simulink model "lab0_model_est"  (R2024b)
settings: Solver=ode45  StartTime=0.0  StopTime=sIn.t_sim  RelTol=1e-3
values from neighbouring files (symbols this model uses):
  PID = computePIDGains(8, 0.15, 0.1, plant.Ps, "PID")    [lab0_startup.m]
undefined symbols (not defined in the file or in its folder): degs2rpm, filt, gbox, rpm2degs, sens, sIn
libraries: simulink x2, simulink_extras x1
settings Model: Creator=pries  LastModifiedBy=pries
settings DataIOCC: ReturnWorkspaceOutputs=off

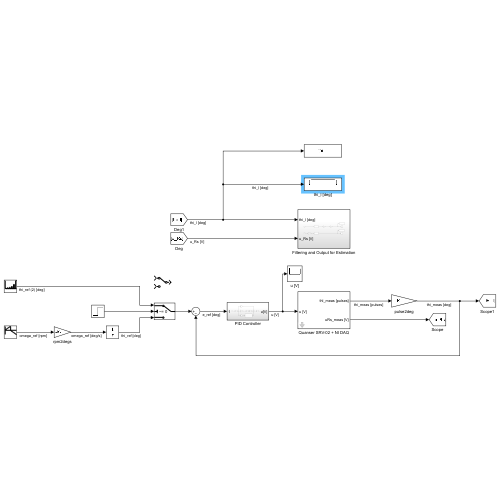
[thumbnail: Simulink's stored preview of the top-level diagram]
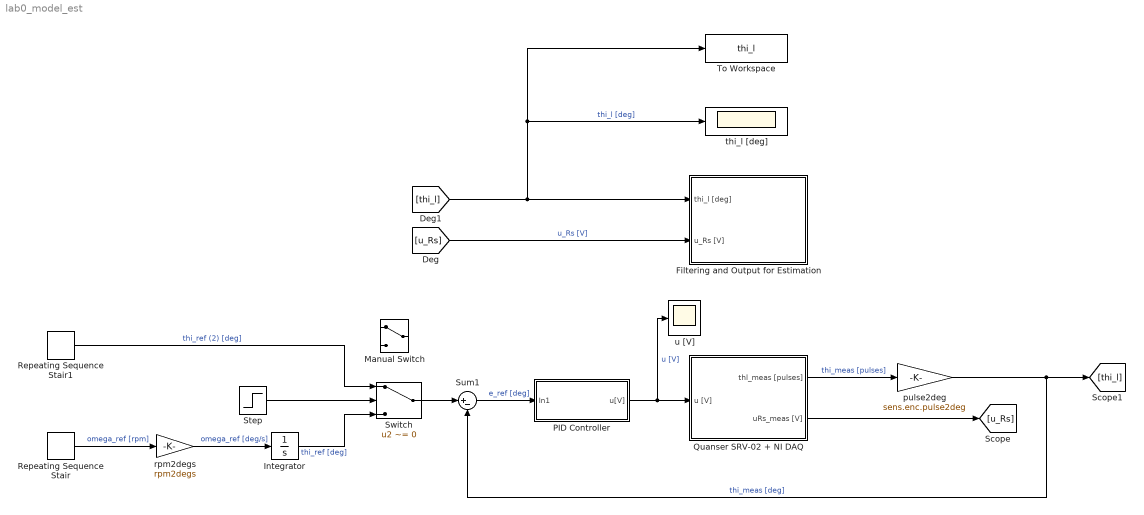
== system lab0_model_est ==
  Filtering and Output for Estimation : Subsystem
  Integrator : Integrator
  Manual Switch : ManualSwitch
  PID Controller : Subsystem
  Quanser SRV-02 + NI DAQ : Subsystem  mask(Quanser SRV-02 (with inertial load) + NI DAQ){Ts=0.001, fricType=Coulomb + viscous}
      mask prompts: Ts "NI DAQ Sample Time:"; fricType "Friction model"
      mask help: Quanser SRV-02 (with inertial load) + NI DAQ model.
      mask init:
      | %%  Sensors data
      | 
      | %   shunt resistor
      | sens.curr.Rs = 0.5;                         %   resistance [Ohm]   
      | sens.curr.uRs_std = 0.01;                   %   voltage noise standard dev [V]                           
      | sens.curr.uRs_var = sens.curr.uRs_std^2;	%   voltage noise variance [V^2]
      | 
      | %   Hewlett-Packard HEDS-5540#A06 optical encoder
      | sens.enc.ppr = 500*4;                       %   pulses per rotation
      | sens.enc.pulse2deg = 360/sens.enc.ppr;      %   [pulses] -> [deg]
      | sens.enc.pulse2rad = 2*pi/sens.enc.ppr;     %   [pulses] -> [rad]
      | sens.enc.deg2pulse = sens.enc.ppr/360;      %   [deg] -> [pulses]
      | sens.enc.rad2pulse = sens.enc.ppr/2/pi;     %   [rad] -> [pulses]
      | 
      | 
      | %%  Data acquisition board (daq) data
      | 
      | %   NI PCI-6221 DAC data
      | daq.dac.bits = 16;                                  %   resolution (bits)
      | daq.dac.fs   = 10;                                  %   full scale 
      | daq.dac.q    = 2*daq.dac.fs/(2^daq.dac.bits-1);     %	quantization
      | 
      | %   NI PCI-6221 ADC data
      | daq.adc.bits = 16;                                  %   resolution (bits)
      | daq.adc.fs   = 10;                                  %   full scale (as set in SLDRT Analog Input block)
      | daq.adc.q    = 2*daq.adc.fs/(2^daq.adc.bits-1);     %   quantization
      mask Help:
      | Riccardo Antonello (antonello@dei.unipd.it)
      | 
      | April 24, 2020
      | 
      | Dept. of Information Engineering, University of Padova
      mask TypeOptions fricType: Coulomb + viscous | Karnopp
  Repeating Sequence Stair : simulink/Sources/Repeating Sequence Stair  OutValues=sIn.omega_l  tsamp=sIn.step_time  OutMin=[]  OutMax=[]  OutDataTypeStr=double  OutputDataTypeScalingMode=double  OutDataType=fixdt(0,8)  ConRadixGroup=Best Precision: Vector-wise  OutScaling=2^-12
  Repeating Sequence Stair1 : simulink/Sources/Repeating Sequence Stair  OutValues=sIn.resp  tsamp=10  OutMin=[]  OutMax=[]  OutDataTypeStr=double  OutputDataTypeScalingMode=double  OutDataType=fixdt(0,8)  ConRadixGroup=Best Precision: Vector-wise  OutScaling=2^-12
  Step : Step  Time=0  After=sIn.pid  SampleTime=0
  Sum1 : Sum  Inputs=|+-
  Switch : Switch  Criteria=u2 ~= 0  SaturateOnIntegerOverflow=off  InputSameDT=off
  To Workspace : ToWorkspace  VariableName=thi_l  SaveFormat=Timeseries  SampleTime=-1
  pulse2deg : Gain  Gain=sens.enc.pulse2deg
  rpm2degs : Gain  Gain=rpm2degs
  thi_l [deg] : Scope
  u [V] : Scope
  wires:
  Quanser SRV-02 + NI DAQ/1(thl_meas [pulses]) -> pulse2deg/1  "thi_meas [pulses]"
  Sum1/1 -> PID Controller/1(In1)  "e_ref [deg]"
  pulse2deg/1 -> Sum1/2, [thi_l]  "thi_meas [deg]"
  Quanser SRV-02 + NI DAQ/2(uRs_meas [V]) -> [u_Rs]
  Repeating Sequence Stair/1 -> rpm2degs/1  "omega_ref [rpm]"
  rpm2degs/1 -> Integrator/1  "omega_ref [deg/s]"
  [thi_l] -> To Workspace/1, thi_l [deg]/1, Filtering and Output for Estimation/1(thi_l [deg])  "thi_l [deg]"
  [u_Rs] -> Filtering and Output for Estimation/2(u_Rs [V])  "u_Rs [V]"
  Switch/1 -> Sum1/1
  PID Controller/1(u[V]) -> u [V]/1, Quanser SRV-02 + NI DAQ/1(u [V])  "u [V]"
  Step/1 -> Switch/2
  Repeating Sequence Stair1/1 -> Switch/1  "thi_ref (2) [deg]"
  Integrator/1 -> Switch/3  "thi_ref [deg]"

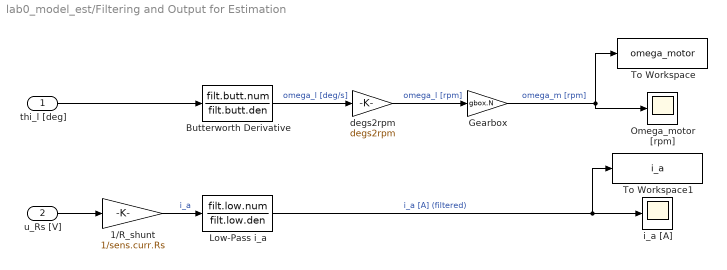
== system lab0_model_est/Filtering and Output for Estimation ==
  thi_l [deg] : Inport
  u_Rs [V] : Inport  Port=2
  1/R_shunt : Gain  Gain=1/sens.curr.Rs
  Butterworth Derivative : TransferFcn  Numerator=filt.butt.num  Denominator=filt.butt.den
  Gearbox : Gain  Gain=gbox.N
  Low-Pass i_a : TransferFcn  Numerator=filt.low.num  Denominator=filt.low.den
  Omega_motor [rpm] : Scope
  To Workspace : ToWorkspace  VariableName=omega_motor  SaveFormat=Timeseries  SampleTime=-1
  To Workspace1 : ToWorkspace  VariableName=i_a  SaveFormat=Timeseries  SampleTime=-1
  degs2rpm : Gain  Gain=degs2rpm
  i_a [A] : Scope
  wires:
  1/R_shunt/1 -> Low-Pass i_a/1  "i_a"
  Gearbox/1 -> To Workspace/1, Omega_motor [rpm]/1  "omega_m [rpm]"
  Butterworth Derivative/1 -> degs2rpm/1  "omega_l [deg/s]"
  degs2rpm/1 -> Gearbox/1  "omega_l [rpm]"
  u_Rs [V]/1 -> 1/R_shunt/1
  Low-Pass i_a/1 -> To Workspace1/1, i_a [A]/1  "i_a [A] (filtered)"
  thi_l [deg]/1 -> Butterworth Derivative/1

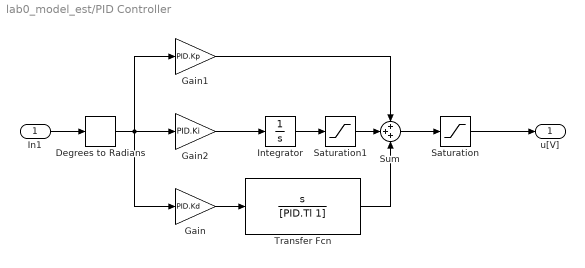
== system lab0_model_est/PID Controller ==
  In1 : Inport
  Degrees to Radians : simulink_extras/Transformations/Degrees to Radians
  Gain : Gain  Gain=PID.Kd
  Gain1 : Gain  Gain=PID.Kp
  Gain2 : Gain  Gain=PID.Ki
  Integrator : Integrator
  Saturation : Saturate  UpperLimit=10  LowerLimit=-10
  Saturation1 : Saturate  UpperLimit=PID.i_saturation  LowerLimit=-PID.i_saturation
  Sum : Sum  Inputs=+++
  Transfer Fcn : TransferFcn  Numerator=[1 0]  Denominator=[PID.Tl 1]
  u[V] : Outport
  wires:
  In1/1 -> Degrees to Radians/1
  Sum/1 -> Saturation/1
  Saturation/1 -> u[V]/1
  Degrees to Radians/1 -> Gain/1, Gain1/1, Gain2/1
  Gain/1 -> Transfer Fcn/1
  Gain2/1 -> Integrator/1
  Transfer Fcn/1 -> Sum/3
  Integrator/1 -> Saturation1/1
  Gain1/1 -> Sum/1
  Saturation1/1 -> Sum/2

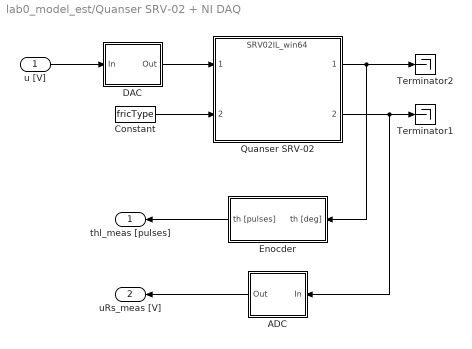
== system lab0_model_est/Quanser SRV-02 + NI DAQ ==
  u [V] : Inport
  ADC : Subsystem
  Constant : Constant  Value=fricType
  DAC : Subsystem
  Enocder : Subsystem
  Quanser SRV-02 : ModelReference  ModelNameDialog=SRV02IL_win64.slxp  ModelReferenceVersion=1.44  CopyOfModelProtected=on
  Terminator1 : Terminator
  Terminator2 : Terminator
  thl_meas [pulses] : Outport
  uRs_meas [V] : Outport  Port=2
  wires:
  Constant/1 -> Quanser SRV-02/2
  Quanser SRV-02/1 -> Terminator2/1, Enocder/1(th [deg])
  u [V]/1 -> DAC/1(In)
  Quanser SRV-02/2 -> Terminator1/1, ADC/1(In)
  DAC/1(Out) -> Quanser SRV-02/1
  ADC/1(Out) -> uRs_meas [V]/1
  Enocder/1(th [pulses]) -> thl_meas [pulses]/1

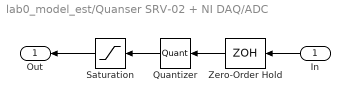
== system lab0_model_est/Quanser SRV-02 + NI DAQ/ADC ==
  In : Inport
  Quantizer : Quantizer  QuantizationInterval=daq.adc.q
  Saturation : Saturate  UpperLimit=daq.adc.fs  LowerLimit=-daq.adc.fs
  Zero-Order Hold : ZeroOrderHold  SampleTime=Ts
  Out : Outport
  wires:
  Zero-Order Hold/1 -> Quantizer/1
  Quantizer/1 -> Saturation/1
  In/1 -> Zero-Order Hold/1
  Saturation/1 -> Out/1

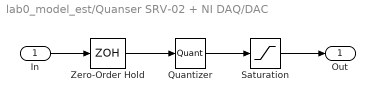
== system lab0_model_est/Quanser SRV-02 + NI DAQ/DAC ==
  In : Inport
  Quantizer : Quantizer  QuantizationInterval=daq.dac.q
  Saturation : Saturate  UpperLimit=daq.dac.fs  LowerLimit=-daq.dac.fs
  Zero-Order Hold : ZeroOrderHold  SampleTime=Ts
  Out : Outport
  wires:
  Saturation/1 -> Out/1
  Zero-Order Hold/1 -> Quantizer/1
  In/1 -> Zero-Order Hold/1
  Quantizer/1 -> Saturation/1

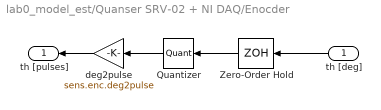
== system lab0_model_est/Quanser SRV-02 + NI DAQ/Enocder ==
  th [deg] : Inport
  Quantizer : Quantizer  QuantizationInterval=sens.enc.pulse2deg
  Zero-Order Hold : ZeroOrderHold  SampleTime=Ts
  deg2pulse : Gain  Gain=sens.enc.deg2pulse
  th [pulses] : Outport
  wires:
  deg2pulse/1 -> th [pulses]/1
  Zero-Order Hold/1 -> Quantizer/1
  th [deg]/1 -> Zero-Order Hold/1
  Quantizer/1 -> deg2pulse/1
